simulink model "Alarm_Switch"  (R2019b)
settings: Solver=VariableStepAuto  StartTime=0.0  StopTime=40  RelTol=1e-3
libraries: dspsnks4 x1, dspvision x1
settings Model: Creator=ARES  LastModifiedBy=ARES
settings SFSimCC: SimAnalyzeCustomCode=on

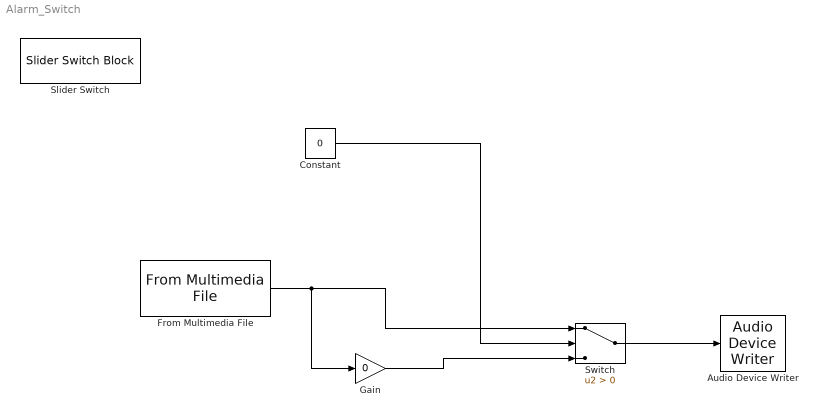
== system Alarm_Switch ==
  Audio Device Writer : dspsnks4/Audio Device Writer  Driver=DirectSound  Device=Default  InheritSampleRate=on  SampleRate=44100  BitDepth=16-bit integer  BufferSize=4096  NumBuffers=10  DefaultOutputChannelMapping=on  OutputChannelMapping=1:2  OutputNumUnderrunSamples=off  DriverIdx=1  DeviceWarnFlag=''
  Constant : Constant  Value=0
  From Multimedia File : dspvision/From Multimedia File  inputFilename=C:\Users\ARES\Documents\ARES Simulation SR\ALARMS\Alarm_Bad.wav  readRange=[1 Inf]  loop=on  numPlays=inf  outputStreams=Audio only  videoDataType=single  audioDataType=double  inheritSampleTime=off  userDefinedSampleTime=1/30  noAudioOutput=off  isIntensityVideo=off  fourcc=RGB  colorVideoFormat=Separate color signals  outputEOF=off  dataOrg=Column-major  audioFrameSize=340  computeAudioFrameSize=off  outSamplingMode=Sample based
      settings: SourceProductName=DSP System Toolbox  SourceProductBaseCode=DS
  Gain : Gain  Gain=0
  Slider Switch : SliderSwitchBlock
      settings: Values={{'Off', 'On'}, [0 1]}
  Switch : Switch  Criteria=u2 > Threshold
  wires:
  Switch/1 -> Audio Device Writer/1
  From Multimedia File/1 -> Gain/1, Switch/1
  Constant/1 -> Switch/2
  Gain/1 -> Switch/3
